simulink library "MyLibrary"  (R2020a)
settings: Solver=VariableStepAuto  StartTime=0.0  StopTime=10.0  RelTol=1e-3
settings Model: Creator=Administrator  LastModifiedBy=Administrator
settings DataIOCC: ReturnWorkspaceOutputs=off
settings DebuggingCC: ArithmeticOperatorsInVariantConditions=warning
settings SFSimCC: SimUseLocalCustomCode=off  CustomCodeUndefinedFunction=UseInterfaceOnly
settings RTWCC: RTWUseLocalCustomCode=off

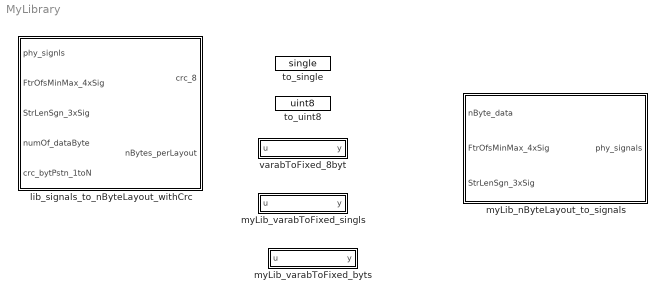
== system MyLibrary ==
  lib_signals_to_nByteLayout_withCrc : Subsystem
  myLib_nByteLayout_to_signals : Subsystem
  myLib_varabToFixed_byts : MATLAB Function  TreatAsAtomicUnit=on
  myLib_varabToFixed_singls : MATLAB Function  TreatAsAtomicUnit=on
  to_single : DataTypeConversion  OutDataTypeStr=single
  to_uint8 : DataTypeConversion  OutDataTypeStr=uint8
  varabToFixed_8byt : MATLAB Function  TreatAsAtomicUnit=on

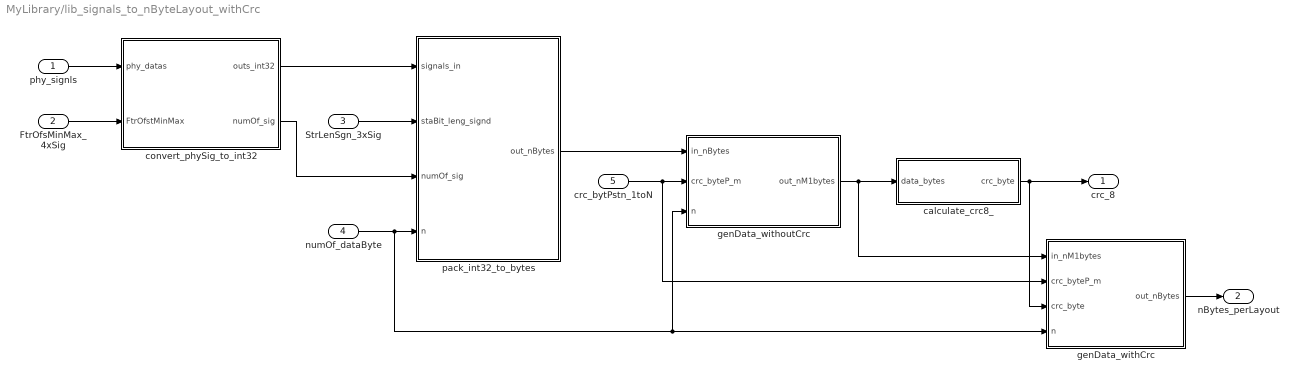
== system MyLibrary/lib_signals_to_nByteLayout_withCrc ==
  phy_signls : Inport  OutDataTypeStr=single
  FtrOfsMinMax_4xSig : Inport  Port=2  OutDataTypeStr=single
  StrLenSgn_3xSig : Inport  Port=3  OutDataTypeStr=uint8
  numOf_dataByte : Inport  Port=4  OutDataTypeStr=uint8  PortDimensions=1
  crc_bytPstn_1toN : Inport  Port=5  OutDataTypeStr=uint8  PortDimensions=1
  calculate_crc8_ : MATLAB Function  TreatAsAtomicUnit=on
  convert_phySig_to_int32 : MATLAB Function  TreatAsAtomicUnit=on
  genData_withCrc : MATLAB Function  TreatAsAtomicUnit=on
  genData_withoutCrc : MATLAB Function  TreatAsAtomicUnit=on
  pack_int32_to_bytes : MATLAB Function  TreatAsAtomicUnit=on
  crc_8 : Outport  OutDataTypeStr=uint8  PortDimensions=1  VectorParamsAs1DForOutWhenUnconnected=off
  nBytes_perLayout : Outport  Port=2  OutDataTypeStr=uint8  VectorParamsAs1DForOutWhenUnconnected=off
  wires:
  FtrOfsMinMax_4xSig/1 -> convert_phySig_to_int32/2(FtrOfstMinMax)
  convert_phySig_to_int32/2(numOf_sig) -> pack_int32_to_bytes/3(numOf_sig)
  calculate_crc8_/1(crc_byte) -> crc_8/1, genData_withCrc/3(crc_byte)
  genData_withCrc/1(out_nBytes) -> nBytes_perLayout/1
  StrLenSgn_3xSig/1 -> pack_int32_to_bytes/2(staBit_leng_signd)
  genData_withoutCrc/1(out_nM1bytes) -> calculate_crc8_/1(data_bytes), genData_withCrc/1(in_nM1bytes)
  crc_bytPstn_1toN/1 -> genData_withoutCrc/2(crc_byteP_m), genData_withCrc/2(crc_byteP_m)
  pack_int32_to_bytes/1(out_nBytes) -> genData_withoutCrc/1(in_nBytes)
  convert_phySig_to_int32/1(outs_int32) -> pack_int32_to_bytes/1(signals_in)
  phy_signls/1 -> convert_phySig_to_int32/1(phy_datas)
  numOf_dataByte/1 -> genData_withoutCrc/3(n), genData_withCrc/4(n), pack_int32_to_bytes/4(n)

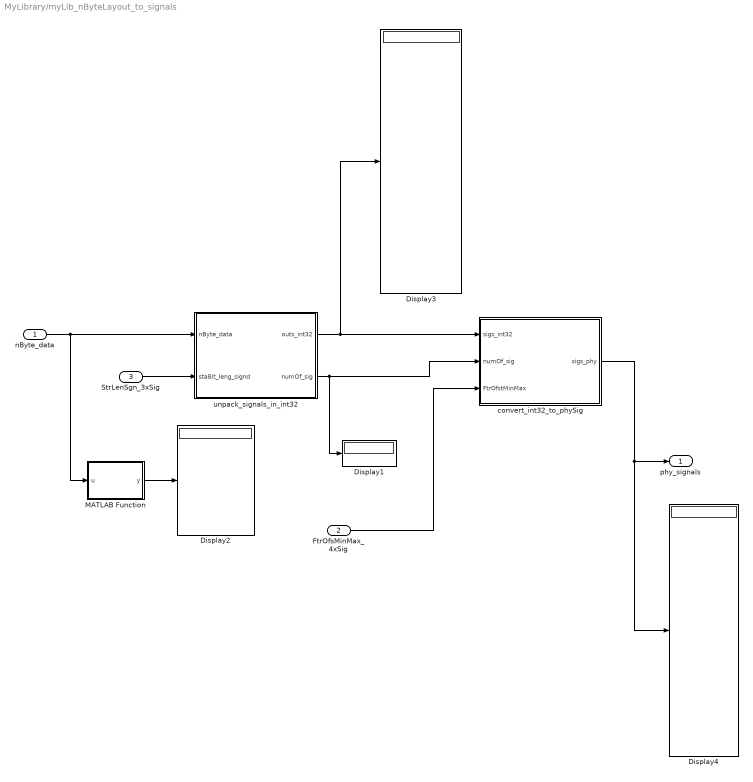
== system MyLibrary/myLib_nByteLayout_to_signals ==
  nByte_data : Inport  OutDataTypeStr=uint8  PortDimensions=8
  FtrOfsMinMax_4xSig : Inport  Port=2  OutDataTypeStr=single
  StrLenSgn_3xSig : Inport  Port=3  OutDataTypeStr=uint8
  Display{1..4} (4 alike) : Display
  MATLAB Function : MATLAB Function  TreatAsAtomicUnit=on
  convert_int32_to_phySig : MATLAB Function  TreatAsAtomicUnit=on
  unpack_signals_in_int32 : MATLAB Function  TreatAsAtomicUnit=on
  phy_signals : Outport
  wires:
  convert_int32_to_phySig/1(sigs_phy) -> phy_signals/1, Display4/1
  FtrOfsMinMax_4xSig/1 -> convert_int32_to_phySig/3(FtrOfstMinMax)
  nByte_data/1 -> MATLAB Function/1(u), unpack_signals_in_int32/1(nByte_data)
  StrLenSgn_3xSig/1 -> unpack_signals_in_int32/2(staBit_leng_signd)
  unpack_signals_in_int32/1(outs_int32) -> Display3/1, convert_int32_to_phySig/1(sigs_int32)
  unpack_signals_in_int32/2(numOf_sig) -> Display1/1, convert_int32_to_phySig/2(numOf_sig)
  MATLAB Function/1(y) -> Display2/1

== matlab function MyLibrary/myLib_varabToFixed_singls ==
  data: u input single size=64; y output single
function y = fcn(u)

fixed_size = 8;
y = single(zeros(fixed_size,1));

for i=1:fixed_size
    y(i) = u(i);
end

== matlab function MyLibrary/varabToFixed_8byt ==
  data: u input uint8 size=8; y output uint8 size=8
function y = fcn(u)

fixed_size = 8;
y = uint8(zeros(fixed_size,1));

for i=1:fixed_size
    y(i) = u(i);
end

== matlab function MyLibrary/myLib_varabToFixed_byts ==
  data: u input uint8 size=8; y output uint8
function y = fcn(u)

fixed_size = 8;
y = uint8(zeros(fixed_size,1));

for i=1:fixed_size
    y(i) = u(i);
end

== matlab function MyLibrary/lib_signals_to_nByteLayout_withCrc/calculate_crc8_ ==
  data: data_bytes input uint8 size=8; crc_byte output uint8 size=1
% function crc8 = fcn(byte_data, bytes)
function crc_byte = fcn(data_bytes)


    t_crc = uint8(hex2dec('ff'));
    [bytes, temp] = size( data_bytes );
    
    for f = 1:bytes
        t_crc = bitxor(data_bytes(f),t_crc);

        for b = 1:8

             if(bitand( t_crc,hex2dec('80') ) ~= 0)  
                   t_crc = bitshift( t_crc,1 );
                   t_crc = bitxor( t_crc,hex2dec('1d') );

             else
                   t_crc = bitshift(t_crc,1);

             end
        end
    end

    %equivalent of c coding: ~t_crc
    crc_byte = bitxor(t_crc, hex2dec('ff'));

== matlab function MyLibrary/lib_signals_to_nByteLayout_withCrc/genData_withCrc ==
  data crc_byteP_m settings: description=start bit, length, signed
  data crc_byte settings: description=start bit, length, signed
  data: in_nM1bytes input uint8; crc_byteP_m input uint8 size=1; out_nBytes output uint8 size=8; crc_byte input uint8 size=1; n input uint8 size=1
function out_nBytes  = fcn(in_nM1bytes, crc_byteP_m, crc_byte, n)

out_nBytes = zeros(n, 1, 'uint8');
in_pstn  = uint8(1);
out_pstn = uint8(1);

while out_pstn <= n   
    if ( out_pstn == crc_byteP_m ) || (0 == crc_byteP_m)  % 0 means no crc is this messagem by convension
        out_nBytes(out_pstn) = crc_byte;   
    else
        out_nBytes(out_pstn) = in_nM1bytes(in_pstn);       
        in_pstn = in_pstn + 1;
    end
    out_pstn = out_pstn + 1;
end 


% if crc_byteP_m == 0   % no crc is this messagem by convension
%     out_nBytes = in_nM1bytes;
%     
% else
%     out_nBytes = zeros(n, 1, 'uint8');
%     in_pstn  = uint8(1);
%     out_pstn = uint8(1);
% 
%     while out_pstn <= n   
%         if out_pstn == crc_byteP_m
%             out_nBytes(out_pstn) = crc_byte;   
%         else
%             out_nBytes(out_pstn) = in_nM1bytes(in_pstn);       
%             in_pstn = in_pstn + 1;
%         end
%         out_pstn = out_pstn + 1;
%     end 
% end

== matlab function MyLibrary/lib_signals_to_nByteLayout_withCrc/genData_withoutCrc ==
  data crc_byteP_m settings: description=start bit, length, signed
  data: in_nBytes input uint8; crc_byteP_m input uint8 size=1; out_nM1bytes output uint8 size=8; n input uint8 size=1
function out_nM1bytes  = fcn(in_nBytes, crc_byteP_m, n)

out_nM1bytes = zeros(n-1,1, 'uint8');

byte_in  = uint8(1);
byte_out = uint8(1);

while byte_in <= n   
    if (byte_in == crc_byteP_m) || (0 == crc_byteP_m)  % 0 means there is no crc in this message
        
    else
        out_nM1bytes(byte_out) = in_nBytes(byte_in);       
        byte_out = byte_out + 1;
    end
    byte_in = byte_in + 1;
end

== matlab function MyLibrary/lib_signals_to_nByteLayout_withCrc/convert_phySig_to_int32 ==
  data FtrOfstMinMax settings: description=factor, offset, min, max
  data: outs_int32 output int32 size=64; phy_datas input single; FtrOfstMinMax input single; numOf_sig output uint8 size=1
function [outs_int32,numOf_sig] = fcn(phy_datas, FtrOfstMinMax)



temp = size(phy_datas);
numOf_sig = uint8(temp(1));

outs_int32 = zeros(numOf_sig, 1, 'int32');

for sig = 1 : numOf_sig 
    in_single = phy_datas(sig);
    i_base = (sig-1) * 4 ;
    factor = FtrOfstMinMax( i_base + 1);
    offset = FtrOfstMinMax( i_base + 2);
    min_v  = FtrOfstMinMax( i_base + 3);
    max_v  = FtrOfstMinMax( i_base + 4);
    
    if (in_single < min_v ) || (in_single > max_v )
        "Error 1319"
    end
    out_int32       = int32( (in_single - offset)/factor );    
    outs_int32(sig) = out_int32;
end

== matlab function MyLibrary/lib_signals_to_nByteLayout_withCrc/pack_int32_to_bytes ==
  data staBit_leng_signd settings: description=start bit, length, signed
  data: signals_in input int32; out_nBytes output uint8 size=8; staBit_leng_signd input uint8; numOf_sig input uint8 size=1; n input uint8 size=1
function out_nBytes = fcn(signals_in, staBit_leng_signd, numOf_sig, n)

out_nBytes = zeros(n, 1, 'uint8');

for sig = 1 : numOf_sig 
    % get data
    data = signals_in(sig);
    strBit =  staBit_leng_signd( (sig-1)*3 + 1 ) + 1; % +1 is because we use matlab counting inside this function
    leng   =  staBit_leng_signd( (sig-1)*3 + 2 );
    signed =  staBit_leng_signd( (sig-1)*3 + 3 );
    
    
    % determine the address (row/byte and column/bit) of the starting bit
%    row_byt = uint8(floor(strBit/uint8(8) ) );
    row_byt = uint8( floor( single(strBit-1)/single(8) ) ) + 1;   % -1 is to start from 0 instead of 1 
%    col_bit = strBit - (row_byt - 1) * 8;  
    col_bit = mod(strBit-1, 8) + 1;   % -1 is to start from 0 instead of 1
    
    % copy each bit in data into the CAN layout
    for bit_i = 1 :1 :leng
      
        if signed && (bit_i == leng)    % special case for signed input and at the msb
            v = bitget(data, 32 );        % msb of the input data int32                    
        else    % all regular case
            v = bitget( data, bit_i );     
        end
        
        out_nBytes(row_byt) = bitset( out_nBytes(row_byt), col_bit, v);
        
        col_bit = col_bit + 1;
        if (col_bit > 8)
            col_bit = uint8(1);
            row_byt = row_byt - 1;   % this is the way layout goes
            
        end
    end
    
    
end

== matlab function MyLibrary/myLib_nByteLayout_to_signals/unpack_signals_in_int32 ==
  data staBit_leng_signd settings: description=start bit, length, signed
  data: outs_int32 output int32 size=64; nByte_data input uint8 size=8; numOf_sig output uint8 size=1; staBit_leng_signd input uint8
function [outs_int32,numOf_sig] = fcn(nByte_data, staBit_leng_signd)



temp = size(staBit_leng_signd);
numOf_sig = uint8(temp(1)/3);

outs_int32 = zeros(numOf_sig, 1, 'int32');


for sig = 1 : numOf_sig 
    outs_int32(sig) = int32(0);
    
    strBit =  staBit_leng_signd( (sig-1)*3 + 1 ) + 1; % +1 is because we use matlab counting inside this function
    leng   =  staBit_leng_signd( (sig-1)*3 + 2 );
    signed =  staBit_leng_signd( (sig-1)*3 + 3 );

    % determine the address (row/byte and column/bit) of the starting bit
    row_byt = uint8( floor( single(strBit-1)/single(8) ) ) + 1;   % -1 is to start from 0 instead of 1 
    col_bit = mod(strBit-1, 8) + 1;   % -1 is to start from 0 instead of 1, lsb position
    byte_data = nByte_data( row_byt ); 
    
    for bit_i = 1 :1 :leng    % extract each bit from lsb to msb
        v = bitget(byte_data, col_bit); 
        outs_int32(sig) = bitset(outs_int32(sig), bit_i ,v);
        
        col_bit = col_bit + 1;
        if col_bit > 8
            row_byt = row_byt -1;   % this is the way layout goes
            col_bit = uint8(1);
            if row_byt > 1   % otherwise, there is nowhere to go
                byte_data = nByte_data( row_byt );   
            end
            
        end
        
    end
    
end

== matlab function MyLibrary/myLib_nByteLayout_to_signals/MATLAB Function ==
  data: u input size=8; y output
function y = fcn(u)

y = size(u);

== matlab function MyLibrary/myLib_nByteLayout_to_signals/convert_int32_to_phySig ==
  data FtrOfstMinMax settings: description=factor, offset, min, max
  data: sigs_int32 input int32 size=64; numOf_sig input uint8 size=1; FtrOfstMinMax input single; sigs_phy output single size=64
function sigs_phy  = fcn(sigs_int32, numOf_sig, FtrOfstMinMax)

sigs_phy = zeros(numOf_sig, 1, 'single');

for sig_i = 1 : numOf_sig 
%   in_single = phy_datas(sig_i);
    i_base = (sig_i-1) * 4 ;
    factor = FtrOfstMinMax( i_base + 1);
    offset = FtrOfstMinMax( i_base + 2);
    min_v  = FtrOfstMinMax( i_base + 3);
    max_v  = FtrOfstMinMax( i_base + 4);

    sigs_phy(sig_i) = single(sigs_int32(sig_i)) * factor + offset;    
    
    if (sigs_phy(sig_i) < min_v ) || (sigs_phy(sig_i) > max_v )
        "Error: exceed min or max value"
    end    

end
